simulink model "mExternalMfileRef"  (Simulink 7.3)
settings: Solver=FixedStepDiscrete  StartTime=0.0  StopTime=10.0  FixedStep=0.2  RelTol=1e-3
settings Model: Creator=yzhan  LastModifiedBy=sbergstr  RecordCoverage=on  CovMetricSettings=dcmtrw  CovModelRefEnable=off  BufferReuse=off
settings OptimizationCC: InlineParams=on  OptimizeBlockIOStorage=off  BufferReuse=off  ExpressionFolding=off  LocalBlockOutputs=off  EfficientMapNaN2IntZero=off

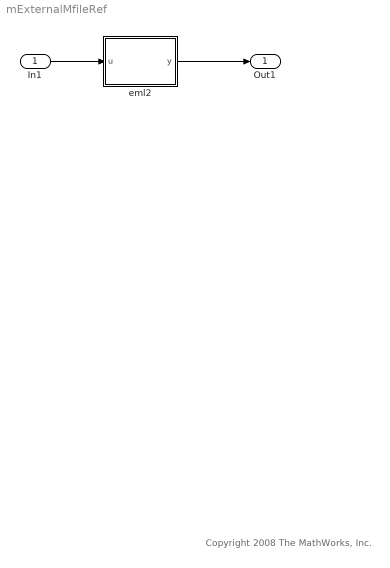
== system mExternalMfileRef ==
  note: Copyright 2008 The MathWorks, Inc.
  In1 : Inport  DataType=double  OutDataType=sfix(16)  OutScaling=2^0  OutDataTypeStr=double
  eml2 : Stateflow chart
  Out1 : Outport  OutDataType=sfix(16)  OutScaling=2^0
  wires:
  In1/1 -> eml2/1(u)
  eml2/1(y) -> Out1/1

== matlab function eml2 ==
  data: u input double; y output double
function y = fcn(u)
% This block supports the Embedded MATLAB subset.
% See the help menu for details. 
b = externalmfile(u);
a = externalmfile1(u);
y =a+u+b+3;
